simulink model "PMRAM"  (R2018a)
settings: Solver=VariableStepAuto  StartTime=0.0  StopTime=1  RelTol=1e-3
libraries: simulink x1
settings Model: Creator=pc  LastModifiedBy=pc

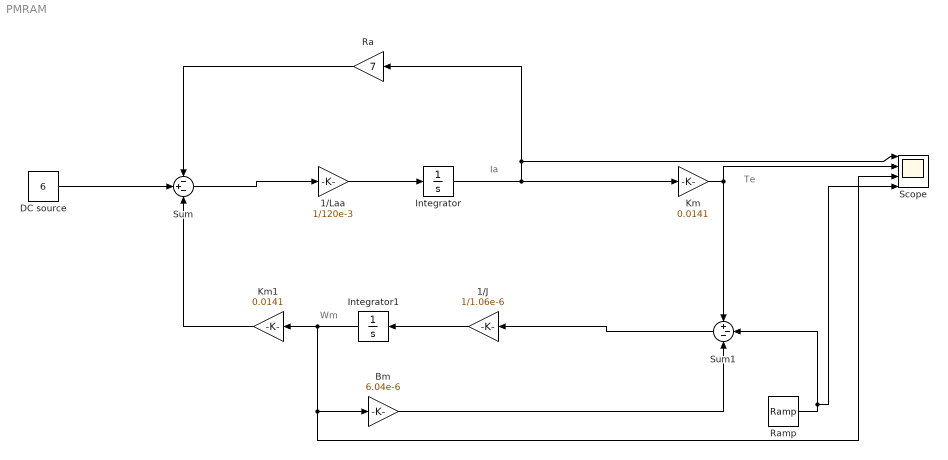
== system PMRAM ==
  note: Ia
  note: Wm
  note: Te
  1/J : Gain  Gain=1/1.06e-6
  1/Laa : Gain  Gain=1/120e-3
  Bm : Gain  Gain=6.04e-6
  DC source : Constant  Value=6
  Integrator : Integrator
  Integrator1 : Integrator
  Km : Gain  Gain=0.0141
  Km1 : Gain  Gain=0.0141
  Ra : Gain  Gain=7
  Ramp : simulink/Sources/Ramp  slope=0.025  start=0.5  InitialOutput=0
  Scope : Scope  NumInputPorts=4
  Sum : Sum  Inputs=-+-
  Sum1 : Sum  Inputs=+--
  wires:
  Integrator/1 -> Scope/1, Ra/1, Km/1
  1/Laa/1 -> Integrator/1
  DC source/1 -> Sum/2
  Bm/1 -> Sum1/3
  Ramp/1 -> Scope/4, Sum1/2
  1/J/1 -> Integrator1/1
  Km/1 -> Sum1/1, Scope/2
  Integrator1/1 -> Km1/1, Scope/3, Bm/1
  Sum/1 -> 1/Laa/1
  Sum1/1 -> 1/J/1
  Ra/1 -> Sum/1
  Km1/1 -> Sum/3
